simulink model "SAR_NS_v1"  (R2019b)
settings: Solver=VariableStepAuto  StartTime=0.0  StopTime=1e-6  RelTol=1e-3
values from neighbouring files (symbols this model uses):
  B = 10    [TB_SAR.m]    (also in TB_SAR_Histogram.m; TB_SAR_NS.m = 8; func_test.m = [4;5])
  fsig = 173e3    (= 173000)    [TB_SAR.m]    (also in TB_SAR_Histogram.m; TB_SAR_NS.m = 23000)
  Tclk = 1/fclk    (= 1e-07)    [TB_SAR.m]    (also in TB_SAR_Histogram.m; TB_SAR_NS.m = 1.5625e-07)
  Tnyq = 1/fnyq    (= 1e-06)    [TB_SAR.m]    (also in TB_SAR_Histogram.m; TB_SAR_NS.m = 1.25e-06)
  vdacn = [ Cn_array(1:B-1) 0]/(sum(Cn_array)+Cp)*vref    [TB_SAR.m]    (also in TB_SAR_Histogram.m = [ Cn_array_mis(1:B-1) 0]/(sum(Cn_array_mis)+Cp)*vfs; TB_SAR_NS.m)
  vdacp = [ Cp_array(1:B-1) 0]/(sum(Cp_array)+Cp)*vref    [TB_SAR.m]    (also in TB_SAR_Histogram.m = [ Cp_array_mis(1:B-1) 0]/(sum(Cp_array_mis)+Cp)*vfs; TB_SAR_NS.m)
  vfs = 2*vref    (= 1.8)    [TB_SAR.m]    (also in TB_SAR_Histogram.m; TB_SAR_NS.m)
  vin_amp = vref*10^(vin_amp_dB/20)    (= 0.849654788657)    [TB_SAR.m]    (also in TB_SAR_Histogram.m = 1.69930957731; TB_SAR_NS.m)
undefined symbols (not defined in the file or in its folder): Amax, cmp_randn_seed, cmp_Var, cmp_Voff, vdac
libraries: dspsigops x48, dspswit3 x1
settings Model: Creator=benve  LastModifiedBy=benve

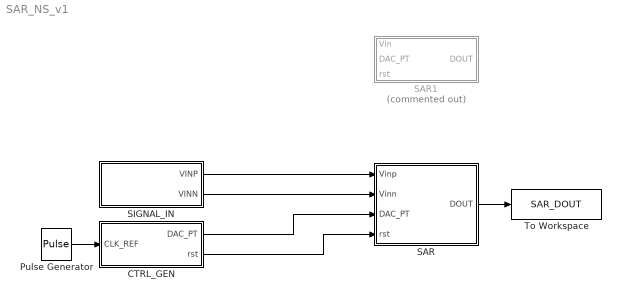
== system SAR_NS_v1 ==
  CTRL_GEN : Subsystem
  Pulse Generator : DiscretePulseGenerator  PulseType=Time based  Amplitude=vfs  Period=Tclk  PulseWidth=50  PhaseDelay=Tclk/2
  SAR : Subsystem
  SAR1 : Subsystem  Commented=on
  SIGNAL_IN : Subsystem
  To Workspace : ToWorkspace  VariableName=SAR_DOUT  SampleTime=-1
  wires:
  Pulse Generator/1 -> CTRL_GEN/1(CLK_REF)
  CTRL_GEN/1(DAC_PT) -> SAR/3(DAC_PT)
  CTRL_GEN/2(rst) -> SAR/4(rst)
  SAR/1(DOUT) -> To Workspace/1
  SIGNAL_IN/2(VINN) -> SAR/2(Vinn)
  SIGNAL_IN/1(VINP) -> SAR/1(Vinp)

== system SAR_NS_v1/CTRL_GEN ==
  CLK_REF : Inport
  Counter : dspswit3/Counter  Direction=Up  CountEvent=Rising edge  CounterSize=User defined  MaxCount=B-1  InitialCount=0  Output=Count and Hit  HitValue=B-1  ResetInput=on  SamplesPerFrame=1  Ts=1  CntDtype=int32  HitDtype=Logical
  Delay1 : Delay  DelayLength=1  InitialCondition=0  SampleTime=Tclk
  Delay3 : Delay  DelayLength=1  InitialCondition=0  SampleTime=Tclk
  DAC_PT : Outport
  rst : Outport  Port=2
  wires:
  Delay1/1 -> rst/1, Counter/2
  Delay3/1 -> DAC_PT/1
  Counter/1 -> Delay3/1
  Counter/2 -> Delay1/1
  CLK_REF/1 -> Counter/1

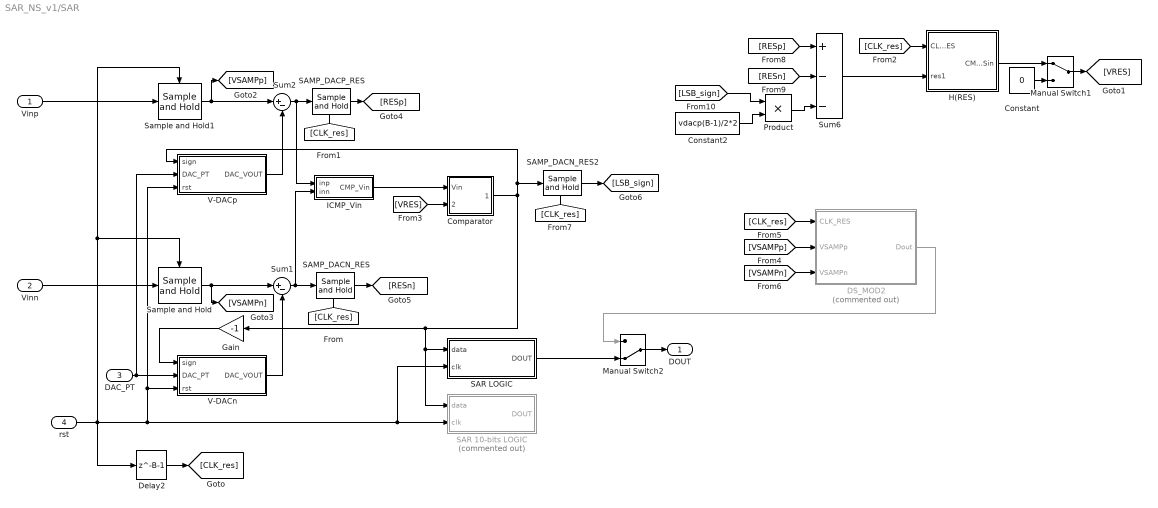
== system SAR_NS_v1/SAR ==
  Vinp : Inport
  Vinn : Inport  Port=2
  DAC_PT : Inport  Port=3
  rst : Inport  Port=4
  Comparator : Subsystem
  Constant : Constant  Value=0
  Constant2 : Constant  Value=vdacp(B-1)/2*2
  DS_MOD2 : Subsystem  Commented=on
  Delay2 : Delay  DelayLength=B-1
  Gain : Gain  Gain=-1
  H(RES) : Subsystem
  ICMP_Vin : Subsystem
  Manual Switch1 : ManualSwitch
  Manual Switch2 : ManualSwitch  CurrentSetting=0
  Product : Product
  SAMP_DACN_RES : dspsigops/Sample and Hold  trig=Rising edge  initCond=0  latchinput=off
  SAMP_DACN_RES2 : dspsigops/Sample and Hold  trig=Rising edge  initCond=0  latchinput=off
  SAMP_DACP_RES : dspsigops/Sample and Hold  trig=Rising edge  initCond=0  latchinput=off
  "SAR 10-bits LOGIC " : Subsystem  Commented=on
  "SAR LOGIC " : Subsystem
  Sample and Hold : dspsigops/Sample and Hold  trig=Rising edge  initCond=0  latchinput=off
  Sample and Hold1 : dspsigops/Sample and Hold  trig=Rising edge  initCond=0  latchinput=off
  Sum1 : Sum  Inputs=|+-
  Sum2 : Sum  Inputs=|+-
  Sum6 : Sum  Inputs=+--
  V-DACn : Subsystem
  V-DACp : Subsystem
  DOUT : Outport
  wires:
  Vinn/1 -> Sample and Hold/1
  V-DACn/1(DAC_VOUT) -> Sum1/2
  DAC_PT/1 -> V-DACn/2(DAC_PT), V-DACp/2(DAC_PT)
  Sample and Hold/1 -> [VSAMPn], Sum1/1
  Vinp/1 -> Sample and Hold1/1
  V-DACp/1(DAC_VOUT) -> Sum2/2
  Sample and Hold1/1 -> [VSAMPp], Sum2/1
  Comparator/1(Sign) -> Gain/1, "SAR LOGIC "/1(data), "SAR 10-bits LOGIC "/1(data), SAMP_DACN_RES2/1, V-DACp/1(sign)
  Sum1/1 -> SAMP_DACN_RES/1, ICMP_Vin/2(inn)
  Sum2/1 -> SAMP_DACP_RES/1, ICMP_Vin/1(inp)
  Gain/1 -> V-DACn/1(sign)
  rst/1 -> Delay2/1, "SAR LOGIC "/2(clk), "SAR 10-bits LOGIC "/2(clk), V-DACn/3(rst), V-DACp/3(rst), Sample and Hold/Trigger, Sample and Hold1/Trigger
  Delay2/1 -> [CLK_res]
  [CLK_res] -> SAMP_DACN_RES/Trigger
  [CLK_res] -> SAMP_DACP_RES/Trigger
  [CLK_res] -> H(RES)/1(CLK_RES)
  H(RES)/1(CMP_RESin) -> Manual Switch1/1
  Manual Switch1/1 -> [VRES]
  Constant/1 -> Manual Switch1/2
  [VRES] -> Comparator/2(RESin)
  ICMP_Vin/1(CMP_Vin) -> Comparator/1(Vin)
  Manual Switch2/1 -> DOUT/1
  "SAR LOGIC "/1(DOUT) -> Manual Switch2/2
  [CLK_res] -> DS_MOD2/1(CLK_RES)
  Sum6/1 -> H(RES)/2(res1)
  [CLK_res] -> SAMP_DACN_RES2/Trigger
  SAMP_DACN_RES2/1 -> [LSB_sign]
  DS_MOD2/1(Dout) -> Manual Switch2/1
  [VSAMPp] -> DS_MOD2/2(VSAMPp)
  [VSAMPn] -> DS_MOD2/3(VSAMPn)
  Product/1 -> Sum6/3
  Constant2/1 -> Product/2
  SAMP_DACP_RES/1 -> [RESp]
  SAMP_DACN_RES/1 -> [RESn]
  [RESp] -> Sum6/1
  [RESn] -> Sum6/2
  [LSB_sign] -> Product/1

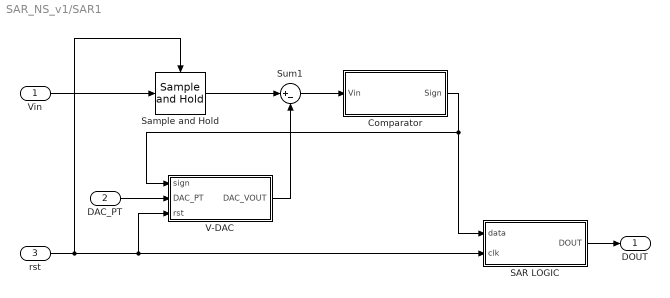
== system SAR_NS_v1/SAR1 ==
  Vin : Inport
  DAC_PT : Inport  Port=2
  rst : Inport  Port=3
  Comparator : Subsystem
  "SAR LOGIC " : Subsystem
  Sample and Hold : dspsigops/Sample and Hold  trig=Rising edge  initCond=0  latchinput=off
  Sum1 : Sum  Inputs=|+-
  V-DAC : Subsystem
  DOUT : Outport
  wires:
  Vin/1 -> Sample and Hold/1
  Comparator/1(Sign) -> V-DAC/1(sign), "SAR LOGIC "/1(data)
  V-DAC/1(DAC_VOUT) -> Sum1/2
  rst/1 -> V-DAC/3(rst), "SAR LOGIC "/2(clk), Sample and Hold/Trigger
  "SAR LOGIC "/1(DOUT) -> DOUT/1
  DAC_PT/1 -> V-DAC/2(DAC_PT)
  Sum1/1 -> Comparator/1(Vin)
  Sample and Hold/1 -> Sum1/1

== system SAR_NS_v1/SIGNAL_IN ==
  Constant : Constant  Value=-1
  Constant1 : Constant
  Product1 : Product
  Product2 : Product
  Sine Wave Function : Sin  Amplitude=vin_amp  Frequency=2*pi*fsig  SampleTime=0
  VINP : Outport
  VINN : Outport  Port=2
  wires:
  Sine Wave Function/1 -> Product1/1, Product2/2
  Constant1/1 -> Product2/1
  Constant/1 -> Product1/2
  Product2/1 -> VINP/1
  Product1/1 -> VINN/1

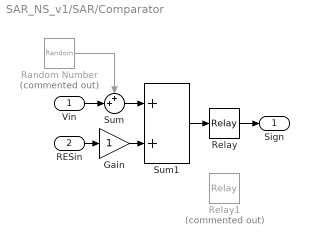
== system SAR_NS_v1/SAR/Comparator ==
  Vin : Inport
  RESin : Inport  Port=2
  Gain : Gain
  Random Number : RandomNumber  Commented=on  Mean=cmp_Voff  Variance=cmp_Var  Seed=cmp_randn_seed  SampleTime=0.1
  Relay : Relay  OffOutputValue=-1
  Relay1 : Relay  Commented=on  OffOutputValue=-1
  Sum : Sum  Inputs=++|
  Sum1 : Sum
  Sign : Outport
  wires:
  Relay/1 -> Sign/1
  Sum1/1 -> Relay/1
  Sum/1 -> Sum1/1
  Vin/1 -> Sum/2
  Random Number/1 -> Sum/1
  RESin/1 -> Gain/1
  Gain/1 -> Sum1/2

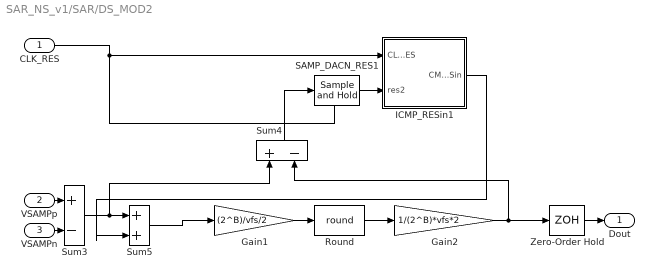
== system SAR_NS_v1/SAR/DS_MOD2 ==
  CLK_RES : Inport
  VSAMPp : Inport  Port=2
  VSAMPn : Inport  Port=3
  Gain1 : Gain  Gain=(2^B)/vfs/2
  Gain2 : Gain  Gain=1/(2^B)*vfs*2
  ICMP_RESin1 : Subsystem
  Round : Rounding  Operator=round
  SAMP_DACN_RES1 : dspsigops/Sample and Hold  trig=Rising edge  initCond=0  latchinput=off
  Sum3 : Sum  Inputs=+-
  Sum4 : Sum  Inputs=+-
  Sum5 : Sum
  Zero-Order Hold : ZeroOrderHold  SampleTime=Tnyq
  Dout : Outport
  wires:
  Gain2/1 -> Sum4/2, Zero-Order Hold/1
  Sum5/1 -> Gain1/1
  Sum3/1 -> Sum4/1, Sum5/1
  Round/1 -> Gain2/1
  ICMP_RESin1/1(CMP_RESin) -> Sum5/2
  Gain1/1 -> Round/1
  Sum4/1 -> SAMP_DACN_RES1/1
  CLK_RES/1 -> SAMP_DACN_RES1/Trigger, ICMP_RESin1/1(CLK_RES)
  VSAMPp/1 -> Sum3/1
  VSAMPn/1 -> Sum3/2
  Zero-Order Hold/1 -> Dout/1
  SAMP_DACN_RES1/1 -> ICMP_RESin1/2(res2)

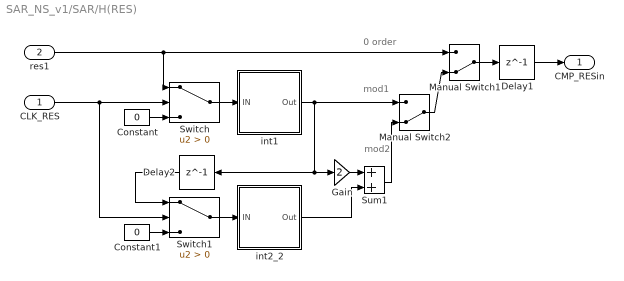
== system SAR_NS_v1/SAR/H(RES) ==
  note: mod1
  note: mod2
  note: 0 order
  CLK_RES : Inport
  res1 : Inport  Port=2
  Constant : Constant  Value=0
  Constant1 : Constant  Value=0
  Delay1 : Delay  DelayLength=1
  Delay2 : Delay  DelayLength=1
  Gain : Gain  Gain=2
  Manual Switch1 : ManualSwitch  CurrentSetting=0
  Manual Switch2 : ManualSwitch  CurrentSetting=0
  Sum1 : Sum
  Switch : Switch  Criteria=u2 > Threshold
  Switch1 : Switch  Criteria=u2 > Threshold
  int1 : Subsystem
  int2_2 : Subsystem
  CMP_RESin : Outport
  wires:
  Manual Switch1/1 -> Delay1/1
  CLK_RES/1 -> Switch1/2, Switch/2
  Switch/1 -> int1/1(IN)
  Constant/1 -> Switch/3
  Delay1/1 -> CMP_RESin/1
  Manual Switch2/1 -> Manual Switch1/2
  int1/1(Out) -> Manual Switch2/1, Gain/1, Delay2/1
  Gain/1 -> Sum1/1
  Sum1/1 -> Manual Switch2/2
  Constant1/1 -> Switch1/3
  Switch1/1 -> int2_2/1(IN)
  int2_2/1(Out) -> Sum1/2
  Delay2/1 -> Switch1/1
  res1/1 -> Manual Switch1/1, Switch/1

== system SAR_NS_v1/SAR/ICMP_Vin ==
  inp : Inport
  inn : Inport  Port=2
  Sum1 : Sum  Inputs=+-
  CMP_Vin : Outport
  wires:
  Sum1/1 -> CMP_Vin/1
  inn/1 -> Sum1/2
  inp/1 -> Sum1/1

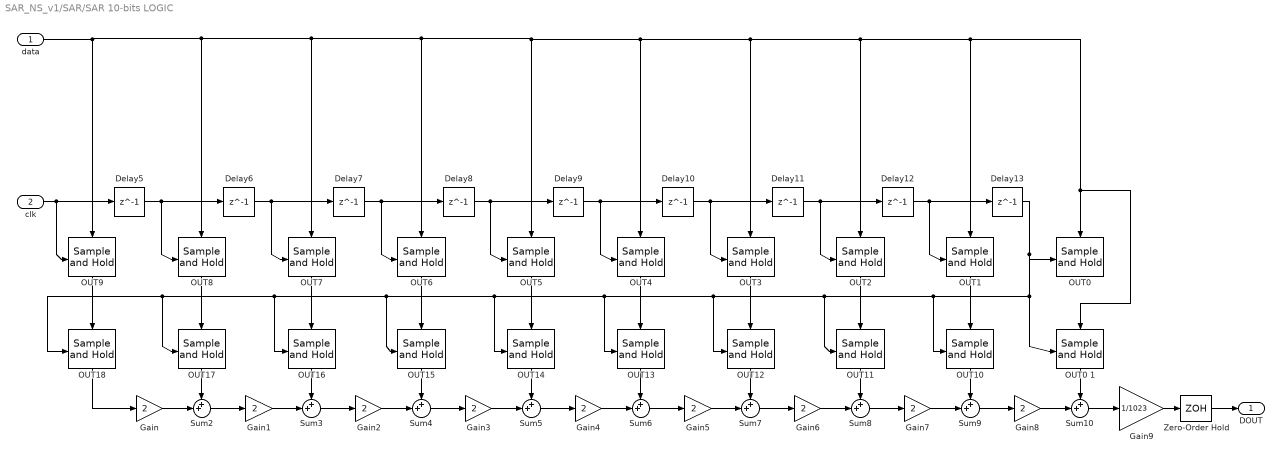
== system SAR_NS_v1/SAR/SAR 10-bits LOGIC  ==
  data : Inport
  clk : Inport  Port=2
  Delay{5..13} (9 alike) : Delay  DelayLength=1  InitialCondition=0  SampleTime=Tclk
  Gain{,1..8} (9 alike) : Gain  Gain=2
  Gain9 : Gain  Gain=1/1023
  "OUT0 " : dspsigops/Sample and Hold  trig=Rising edge  initCond=0  latchinput=off
  OUT0 1 : dspsigops/Sample and Hold  trig=Rising edge  initCond=0  latchinput=off
  OUT{1..18} (18 alike) : dspsigops/Sample and Hold  trig=Rising edge  initCond=0  latchinput=off
  Sum{2..10} (9 alike) : Sum  Inputs=++|
  Zero-Order Hold : ZeroOrderHold  SampleTime=Tnyq
  DOUT : Outport
  wires:
  Sum8/1 -> Gain7/1
  Gain5/1 -> Sum7/2
  Gain/1 -> Sum2/2
  Sum4/1 -> Gain3/1
  Sum3/1 -> Gain2/1
  Delay9/1 -> Delay10/1, OUT4/Trigger
  OUT10/1 -> Sum9/1
  OUT13/1 -> Sum6/1
  Gain1/1 -> Sum3/2
  OUT12/1 -> Sum7/1
  Gain4/1 -> Sum6/2
  OUT14/1 -> Sum5/1
  OUT7/1 -> OUT16/1
  OUT6/1 -> OUT15/1
  Gain2/1 -> Sum4/2
  OUT1/1 -> OUT10/1
  Sum2/1 -> Gain1/1
  OUT9/1 -> OUT18/1
  OUT18/1 -> Gain/1
  Gain3/1 -> Sum5/2
  OUT17/1 -> Sum2/1
  OUT3/1 -> OUT12/1
  OUT8/1 -> OUT17/1
  OUT5/1 -> OUT14/1
  clk/1 -> Delay5/1, OUT9/Trigger
  Delay7/1 -> Delay8/1, OUT6/Trigger
  OUT2/1 -> OUT11/1
  Delay11/1 -> Delay12/1, OUT2/Trigger
  Delay10/1 -> Delay11/1, OUT3/Trigger
  Delay8/1 -> Delay9/1, OUT5/Trigger
  Delay5/1 -> Delay6/1, OUT8/Trigger
  Sum7/1 -> Gain6/1
  Delay6/1 -> Delay7/1, OUT7/Trigger
  Delay13/1 -> "OUT0 "/Trigger, OUT18/Trigger, OUT17/Trigger, OUT16/Trigger, OUT15/Trigger, OUT14/Trigger, OUT13/Trigger, OUT12/Trigger, OUT11/Trigger, OUT10/Trigger, OUT0 1/Trigger
  data/1 -> OUT0 1/1, "OUT0 "/1, OUT1/1, OUT2/1, OUT3/1, OUT4/1, OUT5/1, OUT6/1, OUT7/1, OUT8/1, OUT9/1
  OUT16/1 -> Sum3/1
  Gain9/1 -> Zero-Order Hold/1
  OUT15/1 -> Sum4/1
  Sum5/1 -> Gain4/1
  Gain6/1 -> Sum8/2
  OUT0 1/1 -> Sum10/1
  Gain7/1 -> Sum9/2
  Gain8/1 -> Sum10/2
  OUT4/1 -> OUT13/1
  Sum6/1 -> Gain5/1
  Sum9/1 -> Gain8/1
  Sum10/1 -> Gain9/1
  OUT11/1 -> Sum8/1
  Delay12/1 -> Delay13/1, OUT1/Trigger
  Zero-Order Hold/1 -> DOUT/1

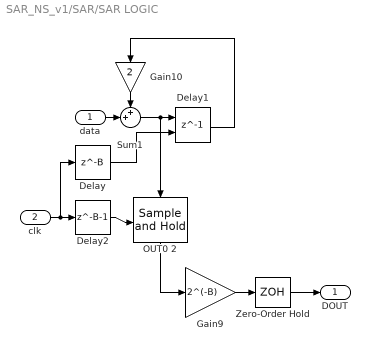
== system SAR_NS_v1/SAR/SAR LOGIC  ==
  data : Inport
  clk : Inport  Port=2
  Delay : Delay  DelayLength=B
  Delay1 : Delay  DelayLength=1  InitialCondition=0  ExternalReset=Rising  SampleTime=Tclk
      settings: InputPortMap=u0,r5
  Delay2 : Delay  DelayLength=B-1
  Gain10 : Gain  Gain=2
  Gain9 : Gain  Gain=2^(-B)
  OUT0 2 : dspsigops/Sample and Hold  trig=Rising edge  initCond=0  latchinput=off
  Sum1 : Sum  Inputs=++|
  Zero-Order Hold : ZeroOrderHold  SampleTime=Tnyq
  DOUT : Outport
  wires:
  Gain9/1 -> Zero-Order Hold/1
  Zero-Order Hold/1 -> DOUT/1
  Gain10/1 -> Sum1/1
  Sum1/1 -> OUT0 2/1, Delay1/1
  Delay1/1 -> Gain10/1
  data/1 -> Sum1/2
  OUT0 2/1 -> Gain9/1
  Delay/1 -> Delay1/2
  clk/1 -> Delay2/1, Delay/1
  Delay2/1 -> OUT0 2/Trigger

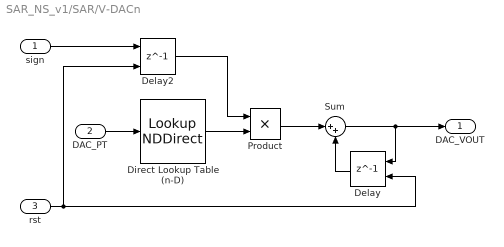
== system SAR_NS_v1/SAR/V-DACn ==
  sign : Inport
  DAC_PT : Inport  Port=2
  rst : Inport  Port=3
  Delay : Delay  DelayLength=1  InitialCondition=0  ExternalReset=Rising  SampleTime=Tclk
      settings: InputPortMap=u0,r5
  Delay2 : Delay  DelayLength=1  InitialCondition=0  ExternalReset=Rising  SampleTime=Tclk
      settings: InputPortMap=u0,r5
  Direct Lookup Table (n-D) : LookupNDDirect  NumberOfTableDimensions=1  Table=vdacn
  Product : Product
  Sum : Sum  Inputs=|++
  DAC_VOUT : Outport
  wires:
  Delay2/1 -> Product/1
  Sum/1 -> DAC_VOUT/1, Delay/1
  rst/1 -> Delay2/2, Delay/2
  Product/1 -> Sum/1
  Delay/1 -> Sum/2
  Direct Lookup Table (n-D)/1 -> Product/2
  DAC_PT/1 -> Direct Lookup Table (n-D)/1
  sign/1 -> Delay2/1

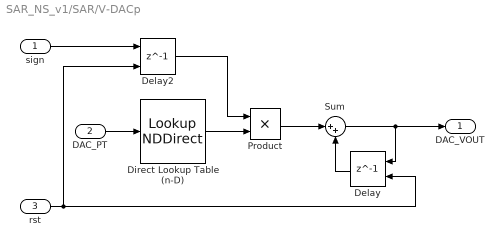
== system SAR_NS_v1/SAR/V-DACp ==
  sign : Inport
  DAC_PT : Inport  Port=2
  rst : Inport  Port=3
  Delay : Delay  DelayLength=1  InitialCondition=0  ExternalReset=Rising  SampleTime=Tclk
      settings: InputPortMap=u0,r5
  Delay2 : Delay  DelayLength=1  InitialCondition=0  ExternalReset=Rising  SampleTime=Tclk
      settings: InputPortMap=u0,r5
  Direct Lookup Table (n-D) : LookupNDDirect  NumberOfTableDimensions=1  Table=vdacp
  Product : Product
  Sum : Sum  Inputs=|++
  DAC_VOUT : Outport
  wires:
  Delay2/1 -> Product/1
  Sum/1 -> DAC_VOUT/1, Delay/1
  rst/1 -> Delay2/2, Delay/2
  Product/1 -> Sum/1
  Delay/1 -> Sum/2
  Direct Lookup Table (n-D)/1 -> Product/2
  DAC_PT/1 -> Direct Lookup Table (n-D)/1
  sign/1 -> Delay2/1

== system SAR_NS_v1/SAR1/Comparator ==
  Vin : Inport
  Relay : Relay  OffOutputValue=-1
  Sign : Outport
  wires:
  Vin/1 -> Relay/1
  Relay/1 -> Sign/1

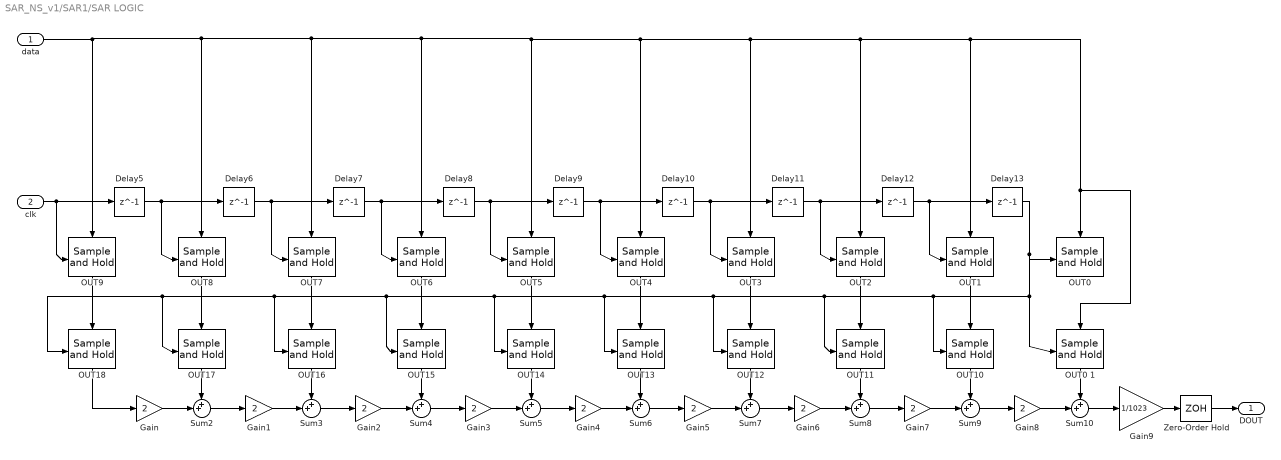
== system SAR_NS_v1/SAR1/SAR LOGIC  ==
  data : Inport
  clk : Inport  Port=2
  Delay{5..13} (9 alike) : Delay  DelayLength=1  InitialCondition=0  SampleTime=1e-9
  Gain{,1..8} (9 alike) : Gain  Gain=2
  Gain9 : Gain  Gain=1/1023
  "OUT0 " : dspsigops/Sample and Hold  trig=Rising edge  initCond=0  latchinput=off
  OUT0 1 : dspsigops/Sample and Hold  trig=Rising edge  initCond=0  latchinput=off
  OUT{1..18} (18 alike) : dspsigops/Sample and Hold  trig=Rising edge  initCond=0  latchinput=off
  Sum{2..10} (9 alike) : Sum  Inputs=++|
  Zero-Order Hold : ZeroOrderHold  SampleTime=1e-9*10
  DOUT : Outport
  wires:
  Sum8/1 -> Gain7/1
  Gain5/1 -> Sum7/2
  Gain/1 -> Sum2/2
  Sum4/1 -> Gain3/1
  Sum3/1 -> Gain2/1
  Delay9/1 -> Delay10/1, OUT4/Trigger
  OUT10/1 -> Sum9/1
  OUT13/1 -> Sum6/1
  Gain1/1 -> Sum3/2
  OUT12/1 -> Sum7/1
  Gain4/1 -> Sum6/2
  OUT14/1 -> Sum5/1
  OUT7/1 -> OUT16/1
  OUT6/1 -> OUT15/1
  Gain2/1 -> Sum4/2
  OUT1/1 -> OUT10/1
  Sum2/1 -> Gain1/1
  OUT9/1 -> OUT18/1
  OUT18/1 -> Gain/1
  Gain3/1 -> Sum5/2
  OUT17/1 -> Sum2/1
  OUT3/1 -> OUT12/1
  OUT8/1 -> OUT17/1
  OUT5/1 -> OUT14/1
  clk/1 -> Delay5/1, OUT9/Trigger
  Delay7/1 -> Delay8/1, OUT6/Trigger
  OUT2/1 -> OUT11/1
  Delay11/1 -> Delay12/1, OUT2/Trigger
  Delay10/1 -> Delay11/1, OUT3/Trigger
  Delay8/1 -> Delay9/1, OUT5/Trigger
  Delay5/1 -> Delay6/1, OUT8/Trigger
  Sum7/1 -> Gain6/1
  Delay6/1 -> Delay7/1, OUT7/Trigger
  Delay13/1 -> "OUT0 "/Trigger, OUT18/Trigger, OUT17/Trigger, OUT16/Trigger, OUT15/Trigger, OUT14/Trigger, OUT13/Trigger, OUT12/Trigger, OUT11/Trigger, OUT10/Trigger, OUT0 1/Trigger
  data/1 -> OUT0 1/1, "OUT0 "/1, OUT1/1, OUT2/1, OUT3/1, OUT4/1, OUT5/1, OUT6/1, OUT7/1, OUT8/1, OUT9/1
  OUT16/1 -> Sum3/1
  Gain9/1 -> Zero-Order Hold/1
  OUT15/1 -> Sum4/1
  Sum5/1 -> Gain4/1
  Gain6/1 -> Sum8/2
  OUT0 1/1 -> Sum10/1
  Gain7/1 -> Sum9/2
  Gain8/1 -> Sum10/2
  OUT4/1 -> OUT13/1
  Sum6/1 -> Gain5/1
  Sum9/1 -> Gain8/1
  Sum10/1 -> Gain9/1
  OUT11/1 -> Sum8/1
  Delay12/1 -> Delay13/1, OUT1/Trigger
  Zero-Order Hold/1 -> DOUT/1

== system SAR_NS_v1/SAR1/V-DAC ==
  sign : Inport
  DAC_PT : Inport  Port=2
  rst : Inport  Port=3
  Delay : Delay  DelayLength=1  InitialCondition=0  ExternalReset=Rising  SampleTime=1e-9
      settings: InputPortMap=u0,r5
  Delay2 : Delay  DelayLength=1  InitialCondition=0  ExternalReset=Rising  SampleTime=1e-9
      settings: InputPortMap=u0,r5
  Direct Lookup Table (n-D) : LookupNDDirect  NumberOfTableDimensions=1  Table=vdac
  Product : Product
  Sum : Sum  Inputs=|++
  DAC_VOUT : Outport
  wires:
  Delay2/1 -> Product/1
  Sum/1 -> DAC_VOUT/1, Delay/1
  rst/1 -> Delay2/2, Delay/2
  Product/1 -> Sum/1
  Delay/1 -> Sum/2
  Direct Lookup Table (n-D)/1 -> Product/2
  DAC_PT/1 -> Direct Lookup Table (n-D)/1
  sign/1 -> Delay2/1

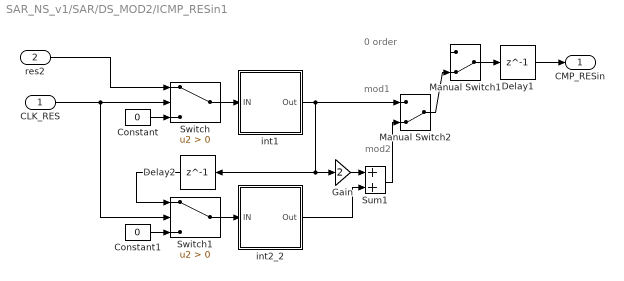
== system SAR_NS_v1/SAR/DS_MOD2/ICMP_RESin1 ==
  note: mod1
  note: mod2
  note: 0 order
  CLK_RES : Inport
  res2 : Inport  Port=2
  Constant : Constant  Value=0
  Constant1 : Constant  Value=0
  Delay1 : Delay  DelayLength=1
  Delay2 : Delay  DelayLength=1
  Gain : Gain  Gain=2
  Manual Switch1 : ManualSwitch  CurrentSetting=0
  Manual Switch2 : ManualSwitch  CurrentSetting=0
  Sum1 : Sum
  Switch : Switch  Criteria=u2 > Threshold
  Switch1 : Switch  Criteria=u2 > Threshold
  int1 : Subsystem
  int2_2 : Subsystem
  CMP_RESin : Outport
  wires:
  Manual Switch1/1 -> Delay1/1
  CLK_RES/1 -> Switch1/2, Switch/2
  Switch/1 -> int1/1(IN)
  Constant/1 -> Switch/3
  Delay1/1 -> CMP_RESin/1
  Manual Switch2/1 -> Manual Switch1/2
  int1/1(Out) -> Manual Switch2/1, Gain/1, Delay2/1
  Gain/1 -> Sum1/1
  Sum1/1 -> Manual Switch2/2
  Constant1/1 -> Switch1/3
  Switch1/1 -> int2_2/1(IN)
  int2_2/1(Out) -> Sum1/2
  Delay2/1 -> Switch1/1
  res2/1 -> Switch/1

== system SAR_NS_v1/SAR/H(RES)/int1 ==
  IN : Inport
  Delay1 : Delay  DelayLength=1  InitialCondition=0
  Gain : Gain
  Saturation : Saturate  Commented=on  UpperLimit=Amax  LowerLimit=-1*Amax
  Sum : Sum  SaturateOnIntegerOverflow=on  InputSameDT=on  OutDataTypeStr=Inherit: Same as first input
  Out : Outport  VectorParamsAs1DForOutWhenUnconnected=off
  wires:
  Sum/1 -> Gain/1
  Gain/1 -> Delay1/1, Out/1
  IN/1 -> Sum/1
  Delay1/1 -> Sum/2

== system SAR_NS_v1/SAR/H(RES)/int2_2 ==
  IN : Inport
  Delay1 : Delay  DelayLength=1  InitialCondition=0
  Gain : Gain
  Saturation : Saturate  Commented=on  UpperLimit=Amax  LowerLimit=-1*Amax
  Sum : Sum  SaturateOnIntegerOverflow=on  InputSameDT=on  OutDataTypeStr=Inherit: Same as first input
  Out : Outport  VectorParamsAs1DForOutWhenUnconnected=off
  wires:
  Sum/1 -> Gain/1
  Gain/1 -> Delay1/1, Out/1
  IN/1 -> Sum/1
  Delay1/1 -> Sum/2

== system SAR_NS_v1/SAR/DS_MOD2/ICMP_RESin1/int1 ==
  IN : Inport
  Delay1 : Delay  DelayLength=1  InitialCondition=0
  Gain : Gain
  Saturation : Saturate  Commented=on  UpperLimit=Amax  LowerLimit=-1*Amax
  Sum : Sum  SaturateOnIntegerOverflow=on  InputSameDT=on  OutDataTypeStr=Inherit: Same as first input
  Out : Outport  VectorParamsAs1DForOutWhenUnconnected=off
  wires:
  Sum/1 -> Gain/1
  Gain/1 -> Delay1/1, Out/1
  IN/1 -> Sum/1
  Delay1/1 -> Sum/2

== system SAR_NS_v1/SAR/DS_MOD2/ICMP_RESin1/int2_2 ==
  IN : Inport
  Delay1 : Delay  DelayLength=1  InitialCondition=0
  Gain : Gain
  Saturation : Saturate  Commented=on  UpperLimit=Amax  LowerLimit=-1*Amax
  Sum : Sum  SaturateOnIntegerOverflow=on  InputSameDT=on  OutDataTypeStr=Inherit: Same as first input
  Out : Outport  VectorParamsAs1DForOutWhenUnconnected=off
  wires:
  Sum/1 -> Gain/1
  Gain/1 -> Delay1/1, Out/1
  IN/1 -> Sum/1
  Delay1/1 -> Sum/2
